simulink model "PV String Partial Shading Model-1"  (R2019b)
settings: Solver=VariableStepAuto  StartTime=0.0  StopTime=1.5  RelTol=1e-6  EnableMultiTasking=on
libraries: powerlib x8, simulink x4, re_lib x4
settings Model: Creator=Rodney Tan  LastModifiedBy=user1
settings DataIOCC: LimitDataPoints=on  SaveFormat=Array  ReturnWorkspaceOutputs=off
settings OptimizationCC: LifeSpan=inf
settings DebuggingCC: SFUnexpectedBacktrackingDiag=warning  SFNoUnconditionalDefaultTransitionDiag=warning  ArithmeticOperatorsInVariantConditions=warning
settings HardwareCC: ProdBitPerPointer=32  ProdBitPerSizeT=32  ProdBitPerPtrDiffT=32  ProdLargestAtomicFloat=None  ProdIntDivRoundTo=Undefined  ProdEndianess=Unspecified  ProdWordSize=32  ProdHWDeviceType=32-bit Generic
settings ModelReferenceCC: PropagateSignalLabelsOutOfModel=off
settings SFSimCC: SimUseLocalCustomCode=off  CustomCodeUndefinedFunction=UseInterfaceOnly
settings RTWCC: RTWUseLocalCustomCode=off
settings CodeAppCC: StateflowObjectComments=on
settings GRTTargetCC: TargetLangStandard=C89/C90 (ANSI)  GeneratePreprocessorConditionals=Disable all
settings ConfigComp: CovMetricSettings=dw  CovHtmlReporting=on  CovSaveCumulativeToWorkspaceVar=on  CovSaveSingleToWorkspaceVar=on  CovExternalEMLEnable=off
settings SimscapeCC: SimscapeNormalizeSystem=off

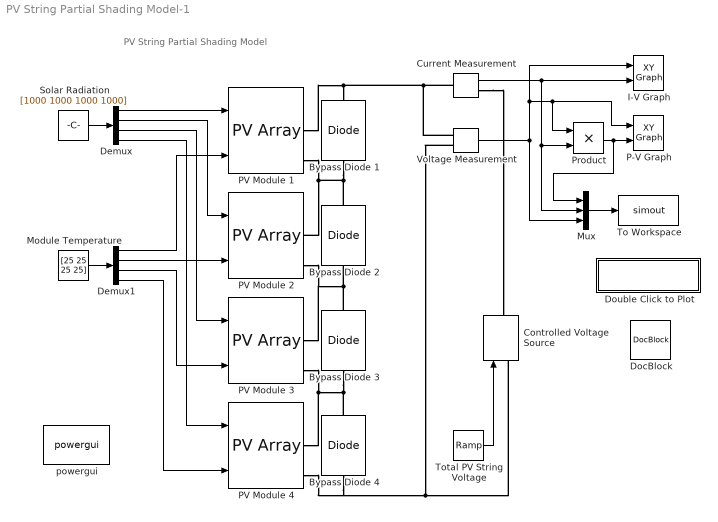
== system PV String Partial Shading Model-1 ==
  note: PV String Partial Shading Model
  Bypass Diode {1..4} (4 alike) : powerlib/Power Electronics/Diode  Ron=0.001  Lon=0  Vf=0.8  IC=0  UseSnubber=off  Rs=500  Cs=250e-9  Measurements=off
      settings: SourceProductName=Simscape Electrical
  Controlled Voltage Source : powerlib/Electrical Sources/Controlled Voltage Source  Initialize=on  Source_Type=DC  Amplitude=0  Phase=0  Frequency=0  Measurements=None
      settings: SourceProductName=Simscape Electrical
  Current Measurement : powerlib/Measurements/Current Measurement  PhasorSimulation=off  OutputType=Complex  PSBequivalent=0
      settings: SourceProductName=Simscape Electrical
  Demux : Demux
  Demux1 : Demux
  DocBlock : simulink/Model-Wide Utilities/DocBlock  DocumentType=Text
      content=|
      | PV String Partial Shading Model
      | Developed by Dr Rodney Tan
      | Version 1.00 (April 2017)
      | This model simulate PV string partial shading and plot its I-V and P-V curve
      |
      | 1. Select your PV Module
      | 2. Set your partial shading profile in the Solar Radiation Block
      | 3. Set the Total PV String Voltage in Ramp Block
      | 4. RUN Simulink
      | 5. Double Click the Plot PV Curve block to plot I-V and P-V curve overlay
  Double Click to Plot : Subsystem
      settings: OpenFcn=PVCurvePlot
      mask Display: disp('Plot PV Curve');
  I-V Graph : simulink/Sinks/XY Graph  xmin=0  xmax=250  ymin=0  ymax=7  st=-1
  Module Temperature : Constant  Value=[25 25 25 25]
  Mux : Mux  Inputs=3
  P-V Graph : simulink/Sinks/XY Graph  xmin=0  xmax=250  ymin=0  ymax=1000  st=-1
  PV Module {1..4} (4 alike) : re_lib/Solar/PV Array  Npar=1  Nser=1  PlotType=array @ 1000 W/m2 & specified temperatures  S_vec="[ 1000  500  100 ]"  Temp_C_vec="[ 45 25  ]"  ModuleName=SunPower SPR-X20-250-BLK  PlotWhenSelected=off  Pm=249.952  Ncell=72  Voc=50.93  Isc=6.2  Vm=42.8  Im=5.84  beta_Voc_pc=-0.35602  alpha_Isc_pc=0.07  beta_Voc=-0.18132  alpha_Isc=0.00434  IL=6.2073  I0=1.8536e-10  nI=1.1367  Rsh=621.2034  Rs=0.301  BAL=off  Tc=1e-6  Tfilter=5e-5
      settings: SourceProductName=Simscape Electrical
  Product : Product
  Solar Radiation : Constant  Value=[1000 1000 1000 1000]
  To Workspace : ToWorkspace  VariableName=simout  SampleTime=-1
  Total PV String Voltage : simulink/Sources/Ramp  slope=210  start=0  InitialOutput=0
  Voltage Measurement : powerlib/Measurements/Voltage Measurement  PhasorSimulation=off  OutputType=Complex  PSBequivalent=0
      settings: SourceProductName=Simscape Electrical
  powergui : powerlib/powergui  Priority=1  SimulationMode=Continuous  SampleTime=50e-6  frequency=60  Iterations=50  frequencyindice=0  Pbase=100e6  ErrMax=1e-4  UnitsV=kV  UnitsW=MW  buscounter=0  FunctionMessages=off  echomessages=off  EnableUseOfTLC=off  CurrentSourceSwitches=off  DisableSnubberDevices=off  DisableRonSwitches=off  DisableVfSwitches=off  DisplayEquations=off  AutomaticDiscreteSolvers=off  SolverType=Tustin/Backward Euler (TBE)  Interpol=off  ExternalGateDelay=off  methode=off  Ts=100  x0status=blocks  SPID=off  SwTol=0  HookPort=off  NonlinearTolerance=0  nMaxIteration=15  ContinueOnMaxIteration=off  RestoreLinks=warning  ResistiveCurrentMeasurement=off  Frange=[0:2:500]  Ylog=off  Xlog=on  ShowGrid=off  save=off  variable=ZData  structure=0  ZoomFFT=off  StartTime=0.0  cycles=1  DisplayStyle=1  fundamental=60  FreqAxis=off  MaxFrequency=1000  frequencyindicesteady=1  RmsSteady=1  display=off
      settings: SourceProductName=Simscape Electrical
  wires:
  Product/1 -> Mux/1, P-V Graph/2
  Total PV String Voltage/1 -> Controlled Voltage Source/1
  Voltage Measurement/1 -> Mux/3, P-V Graph/1, Product/1, I-V Graph/1
  Current Measurement/1 -> I-V Graph/2, Mux/2, Product/2
  Solar Radiation/1 -> Demux/1
  Demux/2 -> PV Module 2/1
  Demux/1 -> PV Module 1/1
  Module Temperature/1 -> Demux1/1
  Demux/3 -> PV Module 3/1
  Demux/4 -> PV Module 4/1
  Demux1/2 -> PV Module 2/2
  Demux1/1 -> PV Module 1/2
  Demux1/3 -> PV Module 3/2
  Demux1/4 -> PV Module 4/2
  Mux/1 -> To Workspace/1
  connections:
  PV Module 3/RConn2 -- Bypass Diode 4/RConn1 -- Bypass Diode 3/LConn1 -- PV Module 4/RConn1
  Bypass Diode 2/RConn1 -- Bypass Diode 1/LConn1 -- PV Module 2/RConn1 -- PV Module 1/RConn2
  Current Measurement/LConn1 -- Voltage Measurement/LConn1 -- PV Module 1/RConn1 -- Bypass Diode 1/RConn1
  Bypass Diode 3/RConn1 -- Bypass Diode 2/LConn1 -- PV Module 2/RConn2 -- PV Module 3/RConn1
  Voltage Measurement/LConn2 -- Controlled Voltage Source/LConn1 -- Bypass Diode 4/LConn1 -- PV Module 4/RConn2
  Current Measurement/RConn1 -- Controlled Voltage Source/RConn1

== system PV String Partial Shading Model-1/Double Click to Plot ==
